simulink model "angular_velocity"  (R2018b)
settings: Solver=FixedStepAuto  StartTime=0.0  StopTime=4.0  FixedStep=.01  RelTol=1e-3
InitFcn:
  | % I_xx=1;
  | % I_yy=2;
  | % I_zz=3;
  | % w_x_0=7;
  | % w_y_0=.2;
  | % w_z_0=.2;
values from neighbouring files (symbols this model uses):
  I_xx = 1    [ps_9_11_7.m]
  I_yy = 2    [ps_9_11_7.m]
  I_zz = 3    [ps_9_11_7.m]
  w_x_0 = 7    [ps_9_11_7.m]
  w_y_0 = .2    (= 0.2)    [ps_9_11_7.m]
  w_z_0 = .2    (= 0.2)    [ps_9_11_7.m]
settings Model: Creator=apollo_liu  LastModifiedBy=apollo_liu

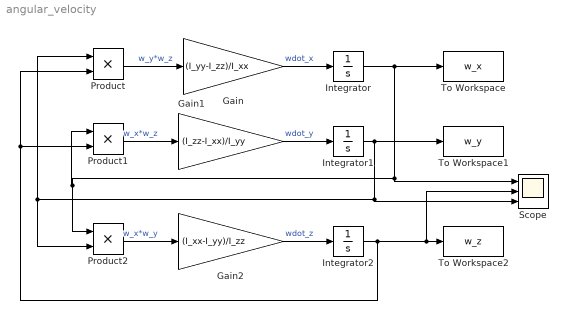
== system angular_velocity ==
  Gain : Gain  Gain=(I_yy-I_zz)/I_xx
  Gain1 : Gain  Gain=(I_zz-I_xx)/I_yy
  Gain2 : Gain  Gain=(I_xx-I_yy)/I_zz
  Integrator : Integrator  InitialCondition=w_x_0
  Integrator1 : Integrator  InitialCondition=w_y_0
  Integrator2 : Integrator  InitialCondition=w_z_0
  Product : Product
  Product1 : Product
  Product2 : Product
  Scope : Scope  NumInputPorts=3
  To Workspace : ToWorkspace  VariableName=w_x  SaveFormat=Timeseries  SampleTime=-1
  To Workspace1 : ToWorkspace  VariableName=w_y  SaveFormat=Timeseries  SampleTime=-1
  To Workspace2 : ToWorkspace  VariableName=w_z  SaveFormat=Timeseries  SampleTime=-1
  wires:
  Gain/1 -> Integrator/1  "wdot_x"
  Product/1 -> Gain/1  "w_y*w_z"
  Gain1/1 -> Integrator1/1  "wdot_y"
  Product1/1 -> Gain1/1  "w_x*w_z"
  Gain2/1 -> Integrator2/1  "wdot_z"
  Product2/1 -> Gain2/1  "w_x*w_y"
  Integrator1/1 -> To Workspace1/1, Scope/3, Product/1, Product2/2
  Integrator2/1 -> To Workspace2/1, Scope/2, Product1/2, Product/2
  Integrator/1 -> To Workspace/1, Scope/1, Product2/1, Product1/1
